simulink library "Solar_Hour_Angle"  (R2018b)
settings: Solver=ode45  StartTime=0.0  StopTime=10.0  RelTol=1e-3  EnableMultiTasking=on
settings Model: Creator=drhf  LastModifiedBy=P41573
settings DataIOCC: LimitDataPoints=on  SaveFormat=Array  SignalLoggingSaveFormat=ModelDataLogs
settings OptimizationCC: ExpressionDepthLimit=2147483647  LifeSpan=inf
settings DebuggingCC: UnderspecifiedInitializationDetection=Classic  MergeDetectMultiDrivingBlocksExec=none  SolverPrmCheckMsg=warning  FcnCallInpInsideContextMsg=warning  StateNameClashWarn=warning  SFUnexpectedBacktrackingDiag=warning  SFNoUnconditionalDefaultTransitionDiag=warning  SFExecutionAtInitializationDiag=none
settings HardwareCC: ProdBitPerPointer=32  ProdBitPerSizeT=32  ProdBitPerPtrDiffT=32  ProdLargestAtomicFloat=None  ProdIntDivRoundTo=Undefined  ProdEndianess=Unspecified  ProdWordSize=32  ProdHWDeviceType=32-bit Generic
settings ModelReferenceCC: PropagateSignalLabelsOutOfModel=off
settings SFSimCC: SimUseLocalCustomCode=off
settings RTWCC: RTWUseLocalCustomCode=off
settings CodeAppCC: StateflowObjectComments=on
settings GRTTargetCC: TargetLangStandard=C89/C90 (ANSI)  GeneratePreprocessorConditionals=Disable all  CombineOutputUpdateFcns=off  GRTInterface=on
settings ConfigComp: CovMetricSettings=dw  CovHtmlReporting=on  CovSaveCumulativeToWorkspaceVar=on  CovSaveSingleToWorkspaceVar=on  CovExternalEMLEnable=off

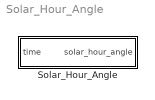
== system Solar_Hour_Angle ==
  Solar_Hour_Angle : Subsystem  mask(Solar Hour Angle){timezone=-15, longitude=-7}
      mask prompts: timezone "longitude of timezone (GMT = 0, east negative) in degree"; longitude "longitude of location (east negative) in degree"
      mask help:
      | The block calls the function "solar_hour_angle" in the CARNOT Library
      | Carlib where the calculation is effectuated.
      | The equation was taken from Duffie, Beckmann: Solar Engineering of
      | Thermal Processes, 2006.
      mask Help: web(fullfile(path_carnot('help'),'Solar_Hour_Angle.html'),'-helpbrowser')

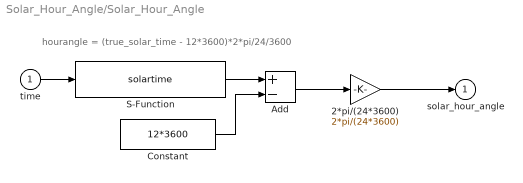
== system Solar_Hour_Angle/Solar_Hour_Angle ==
  note: hourangle = (true_solar_time - 12*3600)*2*pi/24/3600
  time : Inport
  2*pi/(24*3600) : Gain  Gain=2*pi/(24*3600)
  Add : Sum  Inputs=+-
  Constant : Constant  Value=12*3600
  S-Function : S-Function  FunctionName=solartime  Parameters=timezone, longitude  SFunctionDeploymentMode=off  EnableBusSupport=off
  solar_hour_angle : Outport
  wires:
  Constant/1 -> Add/2
  2*pi/(24*3600)/1 -> solar_hour_angle/1
  Add/1 -> 2*pi/(24*3600)/1
  S-Function/1 -> Add/1
  time/1 -> S-Function/1
